simulink model "L7_spring16"  (R2015b)
settings: Solver=VariableStepAuto  StartTime=0.0  StopTime=10.0  RelTol=1e-3
settings Model: Creator=kjartan  LastModifiedBy=kjartan

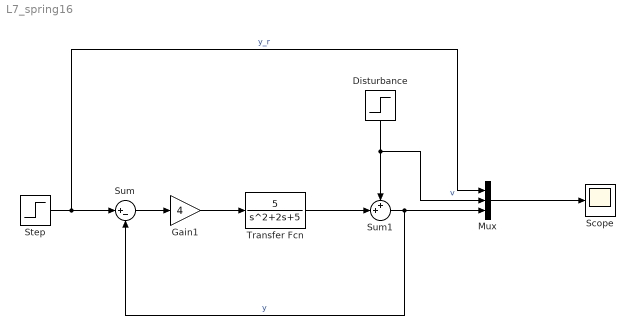
== system L7_spring16 ==
  Disturbance : Step  Time=5  After=-0.5  SampleTime=0
  Gain1 : Gain  Gain=4
  Mux : Mux  Inputs=3
  Scope : Scope
  Step : Step  SampleTime=0
  Sum : Sum  Inputs=|+-
  Sum1 : Sum  Inputs=++|
  Transfer Fcn : TransferFcn  Numerator=[5]  Denominator=[1 2 5]
  wires:
  Mux/1 -> Scope/1
  Transfer Fcn/1 -> Sum1/2
  Step/1 -> Mux/1, Sum/1  "y_r"
  Sum/1 -> Gain1/1
  Gain1/1 -> Transfer Fcn/1
  Sum1/1 -> Sum/2, Mux/3  "y"
  Disturbance/1 -> Sum1/1, Mux/2  "v"
